simulink model "heat_exchanger_PID"  (R2017b)
settings: Solver=VariableStepAuto  StartTime=0.0  StopTime=80  RelTol=1e-3
values from neighbouring files (symbols this model uses):
  Area = n*A_heat_plate    (= 9.8716)    [heat_exchanger_config.m]    (also in linearization.m = 20)
  cp_H2O = 4190    [heat_exchanger_config.m]    (also in linearization.m)
  cp_wort = 4062    [heat_exchanger_config.m]    (also in linearization.m = 4000)
  HE_delay = 25    [heat_exchanger_config.m]    (also in linearization.m = 5)
  m_H2O = m_wort    (= 10)    [heat_exchanger_config.m]    (also in linearization.m = 1)
  m_wort = 10    [heat_exchanger_config.m]    (also in linearization.m = 1)
  T_H2O_in = 5    [heat_exchanger_config.m]    (also in linearization.m = 10)
  T_wort_in = 95    [heat_exchanger_config.m]    (also in linearization.m = 70)
  U = (m_dot_h_data*cp_wort*(T_wort_in-T_wort_out)*log(Delta_T2/Delta_T1))/     (Area*(Delta_T2-Delta_T1))    [heat_exchanger_config.m]    (also in linearization.m = 1000)
libraries: simulink x2
settings Model: PauseTimes=0  Creator=Alexander  LastModifiedBy=Oscar

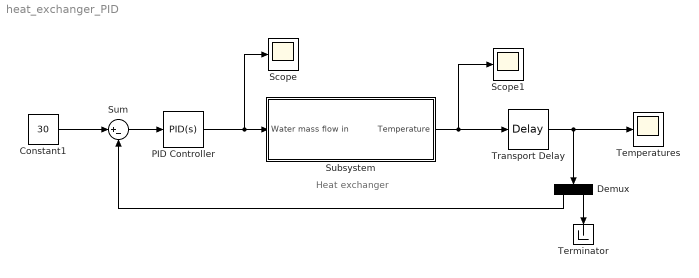
== system heat_exchanger_PID ==
  note: Heat exchanger
  Constant1 : Constant  Value=30
  Demux : Demux  Outputs=2
  PID Controller : simulink/Continuous/PID Controller  Controller=PID  TimeDomain=Continuous-time  SampleTime=-1  IntegratorMethod=Forward Euler  FilterMethod=Forward Euler  Form=Parallel  UseFilter=on  ControllerParametersSource=internal  P=-.25  I=-0.08  D=0.07  N=0.540134521689804  InitialConditionSource=internal  InitialConditionForIntegrator=0  InitialConditionForFilter=0  ExternalReset=none  LimitOutput=on  UpperSaturationLimit=100  LowerSaturationLimit=0  LinearizeAsGain=on  AntiWindupMode=none  Kb=1  TrackingMode=off  Kt=1  PParamMin=[]  PParamMax=[]  IParamMin=[]  IParamMax=[]  DParamMin=[]  DParamMax=[]  NParamMin=[]  NParamMax=[]  KbParamMin=[]  KbParamMax=[]  KtParamMin=[]  KtParamMax=[]  POutMin=[]  POutMax=[]  IOutMin=[]  IOutMax=[]  DOutMin=[]  DOutMax=[]  NOutMin=[]  NOutMax=[]  KbOutMin=[]  KbOutMax=[]  KtOutMin=[]  KtOutMax=[]  IntegratorOutMin=[]  IntegratorOutMax=[]  FilterOutMin=[]  FilterOutMax=[]  SumOutMin=[]  SumOutMax=[]  SumI1OutMin=[]  SumI1OutMax=[]  SumI2OutMin=[]  SumI2OutMax=[]  SumI3OutMin=[]  SumI3OutMax=[]  SumDOutMin=[]  SumDOutMax=[]  SaturationOutMin=[]  SaturationOutMax=[]  IntegratorContinuousStateAttributes=''  IntegratorStateMustResolveToSignalObject=off  IntegratorRTWStateStorageClass=Auto  FilterContinuousStateAttributes=''  FilterStateMustResolveToSignalObject=off  FilterRTWStateStorageClass=Auto  DifferentiatorICPrevScaledInput=0  DifferentiatorOutMin=[]  DifferentiatorOutMax=[]  InitialConditionSetting=State (most efficient)  FilterDiffOutCoefMin=[]  FilterDiffOutCoefMax=[]  SumDenOutMin=[]  SumDenOutMax=[]  SumNumOutMin=[]  SumNumOutMax=[]  ReciprocalOutMin=[]  ReciprocalOutMax=[]  DivideOutMin=[]  DivideOutMax=[]  TunerSelectOption=Transfer Function Based (PID Tuner App)
  Scope : Scope
  Scope1 : Scope
  Subsystem : Subsystem
  Sum : Sum  Inputs=|+-
  Temperatures : Scope
  Terminator : Terminator
  Transport Delay : TransportDelay  DelayTime=HE_delay
  wires:
  Demux/2 -> Terminator/1
  PID Controller/1 -> Scope/1, Subsystem/1(Water mass flow in)
  Transport Delay/1 -> Temperatures/1, Demux/1
  Subsystem/1("Temperature ") -> Transport Delay/1, Scope1/1
  Sum/1 -> PID Controller/1
  Constant1/1 -> Sum/1
  Demux/1 -> Sum/2

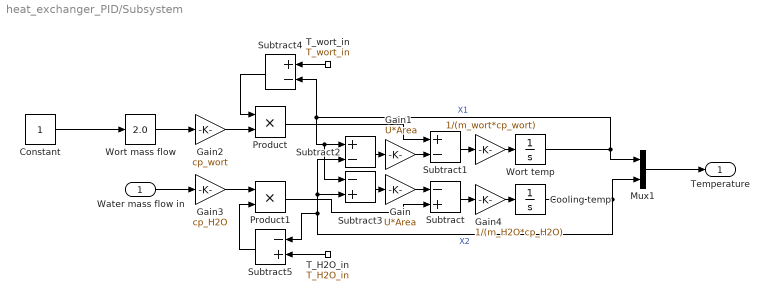
== system heat_exchanger_PID/Subsystem ==
  Water mass flow in : Inport
  " " : Gain  Gain=1/(m_wort*cp_wort)
  Constant : Constant
  Cooling temp : Integrator  InitialCondition=T_H2O_in
  Gain : Gain  Gain=U*Area
  Gain1 : Gain  Gain=U*Area
  Gain2 : Gain  Gain=cp_wort
  Gain3 : Gain  Gain=cp_H2O
  Gain4 : Gain  Gain=1/(m_H2O*cp_H2O)
  Mux1 : Mux  Inputs=2
  Product : Product
  Product1 : Product
  Subtract : Sum  Inputs=-+
  Subtract1 : Sum  Inputs=+-
  Subtract2 : Sum  Inputs=+-
  Subtract3 : Sum  Inputs=-+
  Subtract4 : Sum  Inputs=+-
  Subtract5 : Sum  Inputs=-+
  T_H2O_in : Constant  Value=T_H2O_in
  T_wort_in : Constant  Value=T_wort_in
  Wort mass flow : simulink/Math Operations/Slider Gain  gain=2.0  low=0  high=10
  Wort temp : Integrator  InitialCondition=T_wort_in
  "Temperature " : Outport
  wires:
  Cooling temp/1 -> Subtract5/1, Subtract3/2, Subtract2/2, Mux1/2  "X2"
  Wort temp/1 -> Subtract4/2, Subtract3/1, Subtract2/1, Mux1/1  "X1"
  Mux1/1 -> "Temperature "/1
  Gain1/1 -> Subtract1/2
  Gain/1 -> Subtract/1
  Subtract2/1 -> Gain1/1
  Subtract3/1 -> Gain/1
  " "/1 -> Wort temp/1
  Constant/1 -> Wort mass flow/1
  Subtract1/1 -> " "/1
  Subtract/1 -> Gain4/1
  Gain4/1 -> Cooling temp/1
  T_wort_in/1 -> Subtract4/1
  Wort mass flow/1 -> Gain2/1
  Subtract4/1 -> Product/1
  T_H2O_in/1 -> Subtract5/2
  Gain2/1 -> Product/2
  Product/1 -> Subtract1/1
  Subtract5/1 -> Product1/2
  Gain3/1 -> Product1/1
  Product1/1 -> Subtract/2
  Water mass flow in/1 -> Gain3/1
